simulink model "Single_Phase_Inverter_B"  (R2016a)
settings: Solver=VariableStepAuto  StartTime=0.0  StopTime=0.3  RelTol=1e-3
libraries: powerlib x10, powerlib_meascontrol x1
settings Model: Creator=Rangga  LastModifiedBy=Rangga

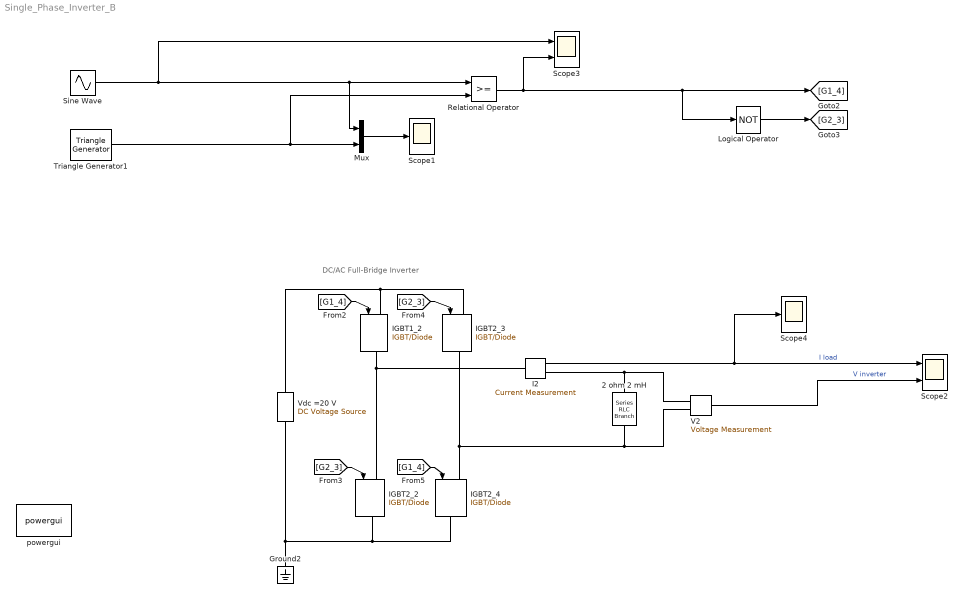
== system Single_Phase_Inverter_B ==
  note: DC/AC Full-Bridge Inverter
  "2 ohm 2 mH " : powerlib/Elements/Series RLC Branch  LConnTagsString=__new0  RConnTagsString=__new0  BranchType=RL  Resistance=2  Inductance=2e-3  SetiL0=off  InitialCurrent=0  Capacitance=[]  Setx0=off  InitialVoltage=0  Measurements=None
  Ground2 : powerlib/Elements/Ground  LConnTagsString=a
  I2 : powerlib/Measurements/Current Measurement  Tag=PoWeRsYsTeMmEaSuReMeNt  PhasorSimulation=off  OutputType=Magnitude  PSBequivalent=0
  IGBT1_2 : powerlib/Power Electronics/IGBT//Diode  Ron=1e-3  Rs=1e5  Cs=inf  Measurements=off
  IGBT2_2 : powerlib/Power Electronics/IGBT//Diode  Ron=1e-3  Rs=1e5  Cs=inf  Measurements=off
  IGBT2_3 : powerlib/Power Electronics/IGBT//Diode  Ron=1e-3  Rs=1e5  Cs=inf  Measurements=off
  IGBT2_4 : powerlib/Power Electronics/IGBT//Diode  Ron=1e-3  Rs=1e5  Cs=inf  Measurements=off
  Logical Operator : Logic  Operator=NOT  AllPortsSameDT=off  OutDataTypeStr=boolean
  Mux : Mux  Inputs=2
  Relational Operator : RelationalOperator  OutDataTypeStr=boolean
  Scope1 : Scope
  Scope2 : Scope  NumInputPorts=2
  Scope3 : Scope  NumInputPorts=2
  Scope4 : Scope
  Sine Wave : Sin  Amplitude=.8  Frequency=2*pi*60  SampleTime=0
  Triangle Generator1 : powerlib_meascontrol/Pulse & Signal Generators/Triangle Generator  Freq=10000  Phase=0  Ts=0
  V2 : powerlib/Measurements/Voltage Measurement  Tag=PoWeRsYsTeMmEaSuReMeNt  PhasorSimulation=off  OutputType=Magnitude  PSBequivalent=0
  Vdc =20 V : powerlib/Electrical Sources/DC Voltage Source  Description=source block  Amplitude=20  Measurements=None
      settings: AttributesFormatString=\n
  powergui : powerlib/powergui  Priority=1  SimulationMode=Continuous  SolverType=Tustin/Backward Euler (TBE)  SampleTime=1e-6  frequency=60  SPID=on  DisableSnubberDevices=off  DisableRonSwitches=off  DisableVfSwitches=off  SwTol=0  DisplayEquations=off  Interpol=off  ExternalGateDelay=off  methode=off  Ts=10  FunctionMessages=off  echomessages=off  HookPort=off  EnableUseOfTLC=off  x0status=blocks  frequencyindice=0  Pbase=100e6  ErrMax=1e-4  Iterations=50  UnitsV=kV  UnitsW=MW  buscounter=0  RestoreLinks=warning  ResistiveCurrentMeasurement=off  Frange=[0:2:500]  Ylog=off  Xlog=on  ShowGrid=off  save=off  variable=ZData  structure=Iout  ZoomFFT=on  StartTime=0.2  cycles=2  DisplayStyle=1  fundamental=60  FreqAxis=off  MaxFrequency=1000  frequencyindicesteady=1  RmsSteady=1  display=off
  wires:
  I2/1 -> Scope4/1, Scope2/1  "I load"
  [G1_4] -> IGBT1_2/1
  [G2_3] -> IGBT2_2/1
  [G2_3] -> IGBT2_3/1
  [G1_4] -> IGBT2_4/1
  Sine Wave/1 -> Scope3/1, Mux/1, Relational Operator/1
  Relational Operator/1 -> Scope3/2, Logical Operator/1, [G1_4]
  Logical Operator/1 -> [G2_3]
  Triangle Generator1/1 -> Mux/2, Relational Operator/2
  Mux/1 -> Scope1/1
  V2/1 -> Scope2/2  "V inverter"
  connections:
  "2 ohm 2 mH "/LConn1 -- V2/LConn1 -- I2/RConn1
  IGBT2_2/RConn1 -- IGBT2_4/RConn1 -- Vdc =20 V/LConn1 -- Ground2/LConn1
  Vdc =20 V/RConn1 -- IGBT1_2/LConn1 -- IGBT2_3/LConn1
  IGBT1_2/RConn1 -- I2/LConn1 -- IGBT2_2/LConn1
  IGBT2_3/RConn1 -- IGBT2_4/LConn1 -- V2/LConn2 -- "2 ohm 2 mH "/RConn1
